simulink model "exp1"  (R2024b)
settings: Solver=VariableStepAuto  StartTime=0.0  StopTime=1  RelTol=1e-3
InitFcn:
  | Voc=32.9;
  | Iscn=8.21;
  | k=1.38e-23;
  | Ns=54;
  | Np=1;
  | G=523;
  | Gn=1000;
  | Kv=-0.1230;
  | Ki=0.0032;
  | T=301;
  | Tn=300;
  | q=1.6e-19;
  | I0n=9.85e-8;
  | Eg=1.12;
  | Ign=8.214;
  | Rs=0.221;
  | Rp=414.5;
  | a=1.0;
libraries: spsSeriesRLCBranchLib x2, spsVoltageMeasurementLib x2, spsControlledCurrentSourceLib x1, spsControlledVoltageSourceLib x1, spsCurrentMeasurementLib x1, simulink x1, sps_lib x1
settings Model: Creator=palla  LastModifiedBy=palla

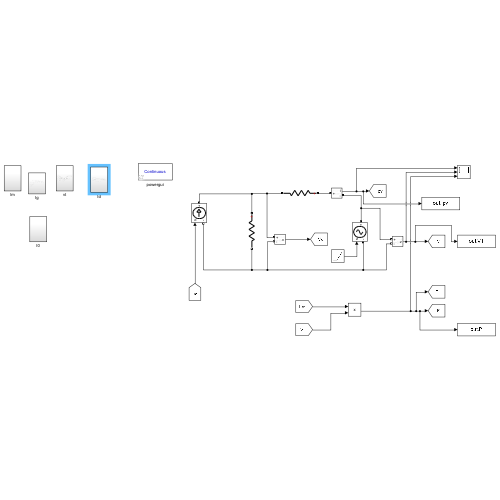
[thumbnail: Simulink's stored preview of the top-level diagram]
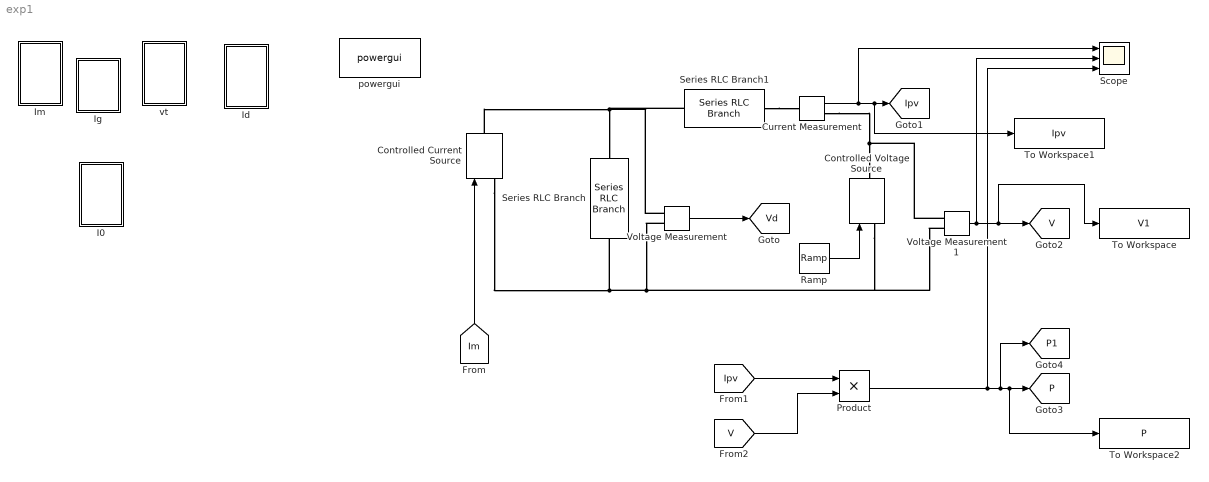
== system exp1 ==
  Controlled Current Source : spsControlledCurrentSourceLib/Controlled Current Source  Initialize=on  Source_Type=AC  Amplitude=0  Phase=0  Frequency=0  Measurements=None
  Controlled Voltage Source : spsControlledVoltageSourceLib/Controlled Voltage Source  Initialize=on  Source_Type=AC  Amplitude=0  Phase=0  Frequency=0  Measurements=None
  Current Measurement : spsCurrentMeasurementLib/Current Measurement  PhasorSimulation=off  OutputType=Complex  PSBequivalent=0
  I0 : Subsystem
  Id : Subsystem
  Ig : Subsystem
  Im : Subsystem
  Product : Product
  Ramp : simulink/Sources/Ramp  slope=32.9  start=0  InitialOutput=0
  Scope : Scope  NumInputPorts=3
  Series RLC Branch : spsSeriesRLCBranchLib/Series RLC Branch  LConnTagsString=__new0  RConnTagsString=__new0  BranchType=R  Resistance=Rp  Inductance=1e-3  SetiL0=off  InitialCurrent=0  Capacitance=1e-6  Setx0=off  InitialVoltage=0  Measurements=None
  Series RLC Branch1 : spsSeriesRLCBranchLib/Series RLC Branch  LConnTagsString=__new0  RConnTagsString=__new0  BranchType=R  Resistance=Rs  Inductance=1e-3  SetiL0=off  InitialCurrent=0  Capacitance=1e-6  Setx0=off  InitialVoltage=0  Measurements=None
  To Workspace : ToWorkspace  VariableName=V1  SampleTime=-1
  To Workspace1 : ToWorkspace  VariableName=Ipv  SampleTime=-1
  To Workspace2 : ToWorkspace  VariableName=P  SampleTime=-1
  Voltage Measurement : spsVoltageMeasurementLib/Voltage Measurement  PhasorSimulation=off  OutputType=Complex  PSBequivalent=0
  Voltage Measurement1 : spsVoltageMeasurementLib/Voltage Measurement  PhasorSimulation=off  OutputType=Complex  PSBequivalent=0
  powergui : sps_lib/powergui  Priority=1  SimulationMode=Continuous  SampleTime=50e-6  frequency=60  Iterations=50  frequencyindice=0  Pbase=100e6  ErrMax=1e-4  UnitsV=kV  UnitsW=MW  buscounter=0  FunctionMessages=off  echomessages=off  EnableUseOfTLC=off  CurrentSourceSwitches=off  DisableSnubberDevices=off  DisableRonSwitches=off  DisableVfSwitches=off  DisplayEquations=off  AutomaticDiscreteSolvers=off  SolverType=Tustin/Backward Euler (TBE)  Interpol=off  ExternalGateDelay=off  methode=off  Ts=100  x0status=blocks  SPID=on  SwTol=0  HookPort=off  NonlinearTolerance=1e-4  nMaxIteration=100  ContinueOnMaxIteration=off  RestoreLinks=warning  ResistiveCurrentMeasurement=off  Frange=[0:2:500]  Ylog=off  Xlog=on  ShowGrid=off  save=off  variable=ZData  structure=0  ZoomFFT=off  StartTime=0.0  cycles=1  DisplayStyle=1  fundamental=60  FreqAxis=off  MaxFrequency=1000  frequencyindicesteady=1  RmsSteady=1  display=off
  vt : Subsystem
  tag scope: Ipv=global, P1=global, P=global, V=global, Vd=global
  wires:
  [Im] -> Controlled Current Source/1
  Voltage Measurement/1 -> [Vd]
  Current Measurement/1 -> Scope/1, To Workspace1/1, [Ipv]
  Ramp/1 -> Controlled Voltage Source/1
  Voltage Measurement1/1 -> Scope/2, To Workspace/1, [V]
  Product/1 -> [P1], To Workspace2/1, [P], Scope/3
  [Ipv] -> Product/1
  [V] -> Product/2
  connections:
  Series RLC Branch1/LConn1 -- Current Measurement/LConn1
  Controlled Current Source/RConn1 -- Voltage Measurement/LConn1 -- Series RLC Branch1/RConn1 -- Series RLC Branch/LConn1
  Controlled Current Source/LConn1 -- Controlled Voltage Source/LConn1 -- Voltage Measurement1/LConn2 -- Voltage Measurement/LConn2 -- Series RLC Branch/RConn1
  Current Measurement/RConn1 -- Voltage Measurement1/LConn1 -- Controlled Voltage Source/RConn1

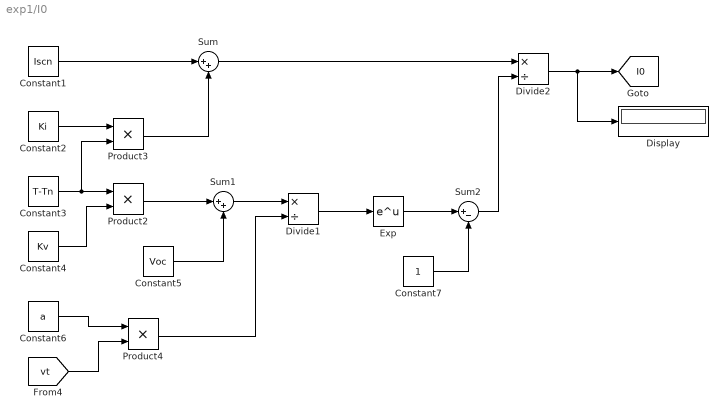
== system exp1/I0 ==
  Constant1 : Constant  Value=Iscn
  Constant2 : Constant  Value=Ki
  Constant3 : Constant  Value=T-Tn
  Constant4 : Constant  Value=Kv
  Constant5 : Constant  Value=Voc
  Constant6 : Constant  Value=a
  Constant7 : Constant
  Display : Display
  Divide1 : Product  Inputs=*/
  Divide2 : Product  Inputs=*/
  Exp : Math
  Product2 : Product
  Product3 : Product
  Product4 : Product
  Sum : Sum  Inputs=|++
  Sum1 : Sum  Inputs=|++
  Sum2 : Sum  Inputs=|+-
  tag scope: I0=global
  wires:
  Constant2/1 -> Product3/1
  Sum/1 -> Divide2/1
  Divide2/1 -> Display/1, [I0]
  Divide1/1 -> Exp/1
  Constant6/1 -> Product4/1
  Sum1/1 -> Divide1/1
  [vt] -> Product4/2
  Product4/1 -> Divide1/2
  Constant4/1 -> Product2/2
  Constant5/1 -> Sum1/2
  Sum2/1 -> Divide2/2
  Constant1/1 -> Sum/1
  Product2/1 -> Sum1/1
  Product3/1 -> Sum/2
  Constant3/1 -> Product3/2, Product2/1
  Exp/1 -> Sum2/1
  Constant7/1 -> Sum2/2

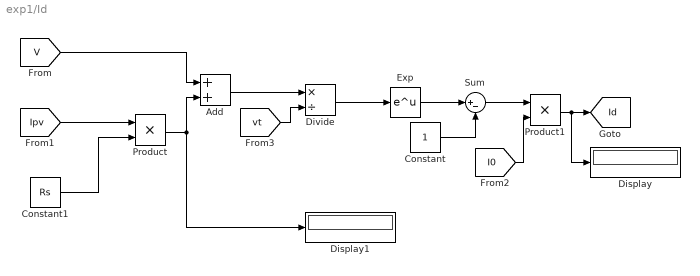
== system exp1/Id ==
  Add : Sum
  Constant : Constant
  Constant1 : Constant  Value=Rs
  Display : Display
  Display1 : Display
  Divide : Product  Inputs=*/
  Exp : Math
  Product : Product
  Product1 : Product
  Sum : Sum  Inputs=|+-
  tag scope: Id=global
  wires:
  Product1/1 -> Display/1, [Id]
  Constant1/1 -> Product/2
  Product/1 -> Add/2, Display1/1
  [I0] -> Product1/2
  [Ipv] -> Product/1
  Exp/1 -> Sum/1
  Constant/1 -> Sum/2
  Sum/1 -> Product1/1
  [V] -> Add/1
  Add/1 -> Divide/1
  [vt] -> Divide/2
  Divide/1 -> Exp/1

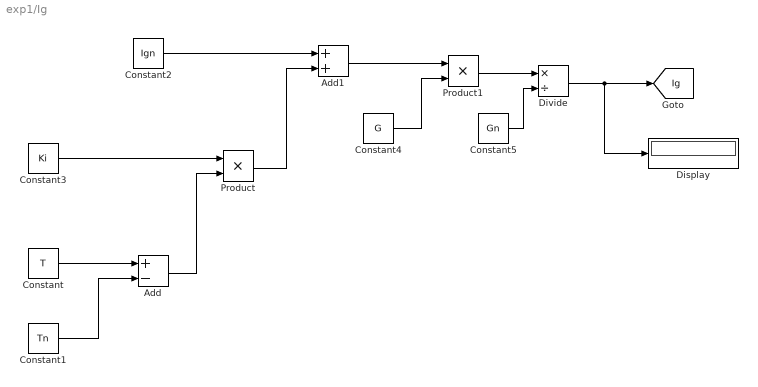
== system exp1/Ig ==
  Add : Sum  Inputs=+-
  Add1 : Sum
  Constant : Constant  Value=T
  Constant1 : Constant  Value=Tn
  Constant2 : Constant  Value=Ign
  Constant3 : Constant  Value=Ki
  Constant4 : Constant  Value=G
  Constant5 : Constant  Value=Gn
  Display : Display
  Divide : Product  Inputs=*/
  Product : Product
  Product1 : Product
  tag scope: Ig=global
  wires:
  Constant2/1 -> Add1/1
  Constant1/1 -> Add/2
  Add/1 -> Product/2
  Constant3/1 -> Product/1
  Add1/1 -> Product1/1
  Constant5/1 -> Divide/2
  Product/1 -> Add1/2
  Constant/1 -> Add/1
  Product1/1 -> Divide/1
  Divide/1 -> Display/1, [Ig]
  Constant4/1 -> Product1/2

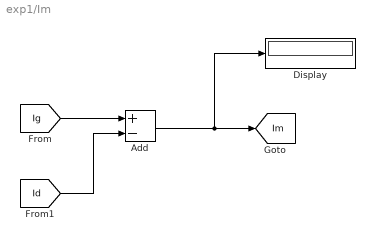
== system exp1/Im ==
  Add : Sum  Inputs=+-
  Display : Display
  tag scope: Im=global
  wires:
  Add/1 -> Display/1, [Im]
  [Id] -> Add/2
  [Ig] -> Add/1

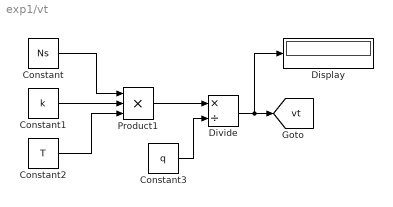
== system exp1/vt ==
  Constant : Constant  Value=Ns
  Constant1 : Constant  Value=k
  Constant2 : Constant  Value=T
  Constant3 : Constant  Value=q
  Display : Display
  Divide : Product  Inputs=*/
  Product1 : Product  Inputs=3
  tag scope: vt=global
  wires:
  Product1/1 -> Divide/1
  Constant3/1 -> Divide/2
  Constant2/1 -> Product1/3
  Constant/1 -> Product1/1
  Divide/1 -> Display/1, [vt]
  Constant1/1 -> Product1/2
